simulink model "Project_Simulink_Section"  (R2023b)
settings: Solver=VariableStepAuto  StartTime=0.0  StopTime=10.0  RelTol=1e-3
libraries: dspfdesign x5, dspmathops x5, dspsnks4 x1, dspvision x1
settings Model: Creator=Azlaan  LastModifiedBy=Azlaan

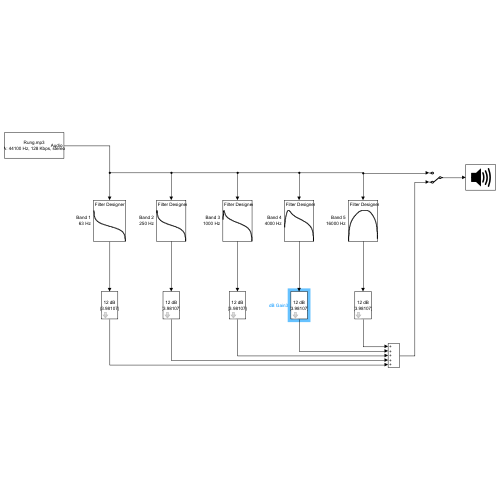
[thumbnail: Simulink's stored preview of the top-level diagram]
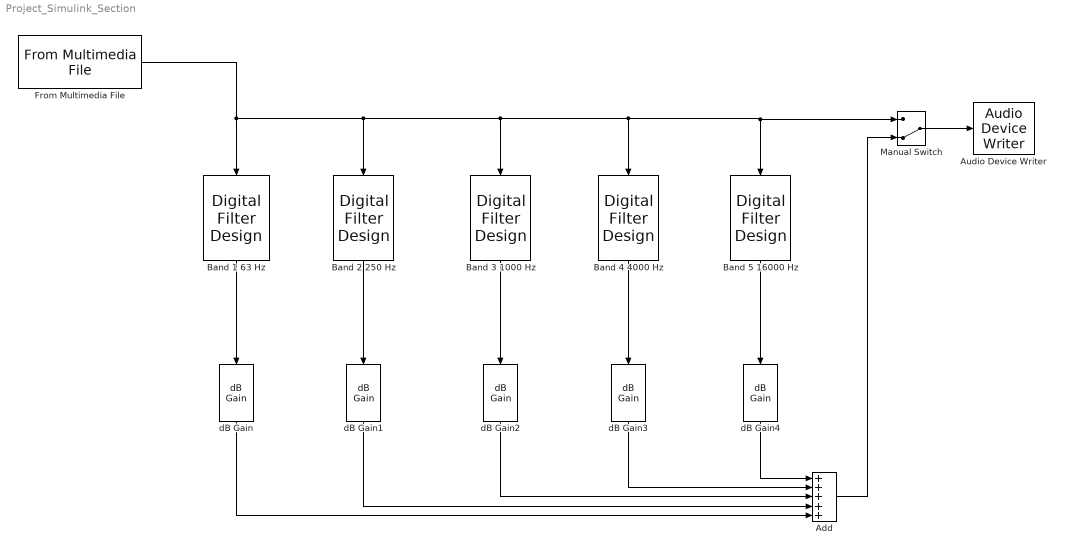
== system Project_Simulink_Section ==
  Add : Sum  Inputs=+++++
  Audio Device Writer : dspsnks4/Audio Device Writer  Driver=DirectSound  Device=Default  InheritSampleRate=on  SampleRate=44100  BitDepth=16-bit integer  BufferSize=4096  NumBuffers=10  DefaultOutputChannelMapping=on  OutputChannelMapping=1:2  OutputNumUnderrunSamples=off  DriverIdx=1  DeviceWarnFlag=''
  Band 1 63 Hz : dspfdesign/Digital Filter Design  mwdsp_browser_bugfix_var=off
  Band 2 250 Hz : dspfdesign/Digital Filter Design  mwdsp_browser_bugfix_var=off
  Band 3 1000 Hz : dspfdesign/Digital Filter Design  mwdsp_browser_bugfix_var=off
  Band 4 4000 Hz : dspfdesign/Digital Filter Design  mwdsp_browser_bugfix_var=off
  Band 5 16000 Hz : dspfdesign/Digital Filter Design  mwdsp_browser_bugfix_var=off
  From Multimedia File : dspvision/From Multimedia File  inputFilename=C:\Users\Azlaan\Music\Rung.mp3  readRange=[1 Inf]  loop=on  numPlays=inf  outputStreams=Audio only  videoDataType=single  audioDataType=double  inheritSampleTime=on  userDefinedSampleTime=1/30  noAudioOutput=off  isIntensityVideo=off  fourcc=RGB  colorVideoFormat=Separate color signals  outputEOF=off  dataOrg=Column-major  audioFrameSize=1024  computeAudioFrameSize=off  outSamplingMode=Sample based
      settings: LibrarySourceBlock=audiosources/From Multimedia File
  Manual Switch : ManualSwitch  CurrentSetting=0
  dB Gain{,1..4} (5 alike) : dspmathops/dB Gain  dB=12  intype=Amplitude
  wires:
  Band 4 4000 Hz/1 -> dB Gain3/1
  Band 5 16000 Hz/1 -> dB Gain4/1
  Band 3 1000 Hz/1 -> dB Gain2/1
  Band 2 250 Hz/1 -> dB Gain1/1
  Band 1 63 Hz/1 -> dB Gain/1
  From Multimedia File/1 -> Manual Switch/1, Band 5 16000 Hz/1, Band 4 4000 Hz/1, Band 3 1000 Hz/1, Band 2 250 Hz/1, Band 1 63 Hz/1
  dB Gain4/1 -> Add/1
  dB Gain3/1 -> Add/2
  dB Gain2/1 -> Add/3
  dB Gain1/1 -> Add/4
  dB Gain/1 -> Add/5
  Add/1 -> Manual Switch/2
  Manual Switch/1 -> Audio Device Writer/1
